simulink model "PID_Motor_control"  (R2015b)
settings: Solver=VariableStepAuto  StartTime=0.0  StopTime=10.0  RelTol=1e-3
libraries: simulink x1
settings Model: Creator=wafiq  LastModifiedBy=wafiq

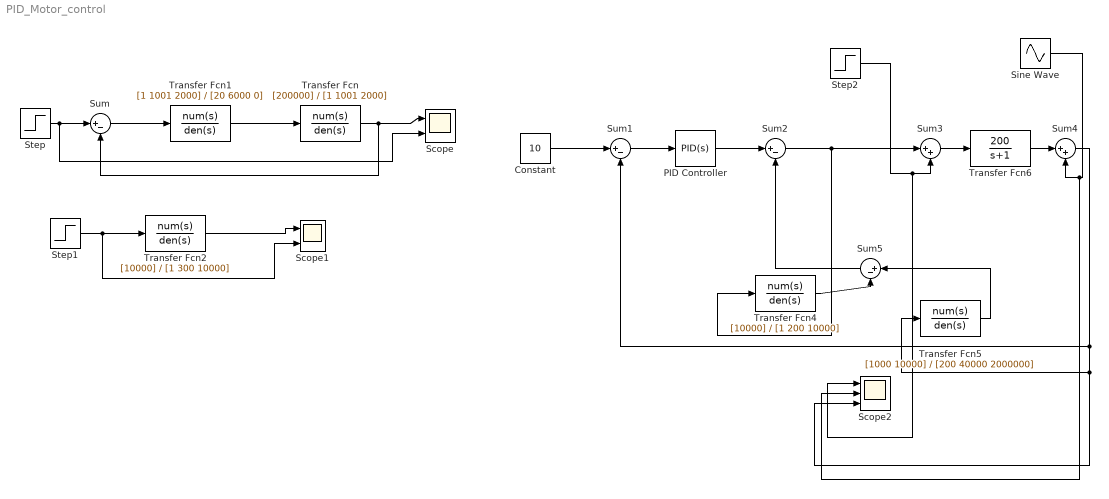
== system PID_Motor_control ==
  Constant : Constant  Value=10  SampleTime=0.5
  PID Controller : simulink/Continuous/PID Controller  Controller=PID  TimeDomain=Continuous-time  SampleTime=-1  IntegratorMethod=Forward Euler  FilterMethod=Forward Euler  Form=Parallel  UseFilter=on  ControllerParametersSource=internal  P=4  I=7.5  D=0.51  N=100  InitialConditionSource=internal  InitialConditionForIntegrator=0  InitialConditionForFilter=0  ExternalReset=none  LimitOutput=off  UpperSaturationLimit=inf  LowerSaturationLimit=-inf  LinearizeAsGain=on  AntiWindupMode=none  Kb=1  TrackingMode=off  Kt=1  PParamMin=[]  PParamMax=[]  IParamMin=[]  IParamMax=[]  DParamMin=[]  DParamMax=[]  NParamMin=[]  NParamMax=[]  KbParamMin=[]  KbParamMax=[]  KtParamMin=[]  KtParamMax=[]  POutMin=[]  POutMax=[]  IOutMin=[]  IOutMax=[]  DOutMin=[]  DOutMax=[]  NOutMin=[]  NOutMax=[]  KbOutMin=[]  KbOutMax=[]  KtOutMin=[]  KtOutMax=[]  IntegratorOutMin=[]  IntegratorOutMax=[]  FilterOutMin=[]  FilterOutMax=[]  SumOutMin=[]  SumOutMax=[]  SumI1OutMin=[]  SumI1OutMax=[]  SumI2OutMin=[]  SumI2OutMax=[]  SumI3OutMin=[]  SumI3OutMax=[]  SumDOutMin=[]  SumDOutMax=[]  SaturationOutMin=[]  SaturationOutMax=[]  IntegratorContinuousStateAttributes=''  IntegratorStateMustResolveToSignalObject=off  IntegratorRTWStateStorageClass=Auto  FilterContinuousStateAttributes=''  FilterStateMustResolveToSignalObject=off  FilterRTWStateStorageClass=Auto  DifferentiatorICPrevScaledInput=0  DifferentiatorOutMin=[]  DifferentiatorOutMax=[]
  Scope : Scope  NumInputPorts=2
  Scope1 : Scope  NumInputPorts=2
  Scope2 : Scope  NumInputPorts=3
  Sine Wave : Sin  Frequency=35/6.2*3.14  SampleTime=0
  Step : Step  SampleTime=0
  Step1 : Step  SampleTime=0
  Step2 : Step  SampleTime=1
  Sum{,1..2,5} (4 alike) : Sum  Inputs=|+-
  Sum3 : Sum  Inputs=|++
  Sum4 : Sum  Inputs=|++
  Transfer Fcn : TransferFcn  Numerator=[200000]  Denominator=[1 1001 2000]
  Transfer Fcn1 : TransferFcn  Numerator=[1 1001 2000]  Denominator=[20 6000 0]
  Transfer Fcn2 : TransferFcn  Numerator=[10000]  Denominator=[1 300 10000]
  Transfer Fcn4 : TransferFcn  Numerator=[10000]  Denominator=[1 200 10000]
  Transfer Fcn5 : TransferFcn  Numerator=[1000 10000]  Denominator=[200 40000 2000000]
  Transfer Fcn6 : TransferFcn  Numerator=[200]  Denominator=[1 1]
  wires:
  Transfer Fcn/1 -> Sum/2, Scope/1
  Step/1 -> Scope/2, Sum/1
  Step1/1 -> Scope1/2, Transfer Fcn2/1
  Transfer Fcn2/1 -> Scope1/1
  Sum/1 -> Transfer Fcn1/1
  Transfer Fcn1/1 -> Transfer Fcn/1
  Transfer Fcn6/1 -> Sum4/1
  Sum2/1 -> Transfer Fcn4/1, Sum3/1
  Sum1/1 -> PID Controller/1
  Constant/1 -> Sum1/1
  PID Controller/1 -> Sum2/1
  Sum4/1 -> Transfer Fcn5/1, Scope2/3, Sum1/2
  Step2/1 -> Scope2/1, Sum3/2
  Sum5/1 -> Sum2/2
  Sine Wave/1 -> Scope2/2, Sum4/2
  Transfer Fcn4/1 -> Sum5/2
  Transfer Fcn5/1 -> Sum5/1
  Sum3/1 -> Transfer Fcn6/1
